simulink model "delay_complex_slr_test"  (Simulink 7.0)
settings: Solver=VariableStepDiscrete  StartTime=0.0  StopTime=500  RelTol=1e-3
libraries: xbsIndex_r4 x7, casper_library x6
settings Model: Creator=User  LastModifiedBy=User
settings DebuggingCC: SaveWithDisabledLinksMsg=none  SaveWithParameterizedLinksMsg=none

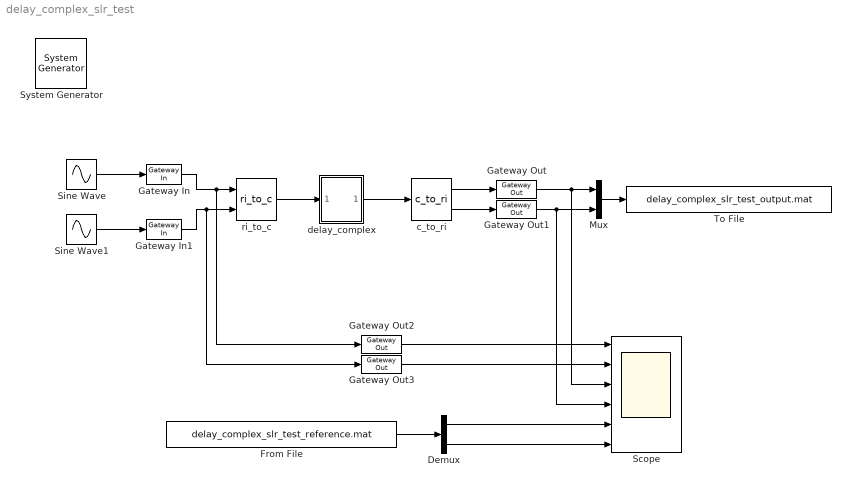
== system delay_complex_slr_test ==
  " System Generator" : xbsIndex_r4/ System Generator  Tag=genX  SystemSampleTime=-1  xilinxfamily=Virtex4  part=xc4vsx35  speed=-10  package=ff668  synthesis_tool=XST  clock_wrapper=Clock Enables  directory=./netlist  testbench=off  simulink_period=1  sysclk_period=100  dcm_input_clock_period=100  incr_netlist=off  trim_vbits=Everywhere in SubSystem  dbl_ovrd=According to Block Masks  core_generation=According to Block Masks  run_coregen=off  deprecated_control=off  eval_field=0  block_type=sysgen
      settings: block_version=10.1.1
  Demux : Demux  Outputs=2
  From File : FromFile  FileName=delay_complex_slr_test_reference.mat  SampleTime=1
  Gateway In : xbsIndex_r4/Gateway In  arith_type="Signed  (2's comp)"  n_bits=13  bin_pt=12  quantization=Truncate  overflow=Wrap  period=1  dbl_ovrd=off  timing_constraint=None  locs_specified=off  LOCs={}  block_type=gatewayin
      settings: infoedit="Gateway in block.  Converts inputs of type Simulink integer, double and fixed point to  Xilinx fixed point type.<P><P>Hardware notes:  In hardware these blocks become top level input ports."  block_version=10.1.1
  Gateway In1 : xbsIndex_r4/Gateway In  arith_type="Signed  (2's comp)"  n_bits=13  bin_pt=12  quantization=Truncate  overflow=Wrap  period=1  dbl_ovrd=off  timing_constraint=None  locs_specified=off  LOCs={}  block_type=gatewayin
      settings: infoedit="Gateway in block.  Converts inputs of type Simulink integer, double and fixed point to  Xilinx fixed point type.<P><P>Hardware notes:  In hardware these blocks become top level input ports."  block_version=10.1.1
  Gateway Out{,1..3} (4 alike) : xbsIndex_r4/Gateway Out  hdl_port=on  timing_constraint=None  locs_specified=off  LOCs={}  block_type=gatewayout
      settings: infoedit="Gateway out block.  Converts Xilinx fixed point inputs into ouputs of type Simulink integer, double, or fixed point.<P><P>Hardware notes:  In hardware these blocks become top level output ports or are discarded, depending on how they are configured."  block_version=10.1.1
  Mux : Mux  Inputs=2
  Scope : Scope  NumInputPorts=6
      settings: YMin=-5~-5~-5~-5~-5~-5  YMax=5~5~5~5~5~5
  Sine Wave : Sin  SineType=Sample based  SampleTime=1
  Sine Wave1 : Sin  SineType=Sample based  Samples=11  SampleTime=1  Offset=10
  To File : ToFile  Filename=delay_complex_slr_test_output.mat  MatrixName=output
  c_to_ri : casper_library/Misc/c_to_ri  SystemSampleTime=-1  n_bits=13  bin_pt=12
      settings: AttributesFormatString=13_12 r/i
  delay_complex : Subsystem  AncestorBlock=casper_library/Delays/delay_complex  mask(delay_complex){delay=7, n_bits=13, bin_pt=12, use_bram=0, bram_latency=4}
      mask prompts: delay "Delay Length"; n_bits "Sample Bit Width"; bin_pt "Binary Point"; use_bram "Use BRAM (0=no, 1=yes)"; bram_latency "BRAM Latency"
      mask help: A delay block that treats its input as complex, splits it into real and imaginary components, delays each component by a specified amount, and then re-joins them into a complex output. The underlying storage is user-selectable (either BRAM or SLR16 elements). The reason for this is wide (36 bit) delays make adjacent multipliers in multiplier-bram pairs unusable.
      mask init:
      | delay_complex_init(gcb, ...
      |     'delay', delay, ...
      |     'n_bits', n_bits, ...
      |     'bin_pt', bin_pt, ...
      |     'use_bram', use_bram, ...
      |     'bram_latency', bram_latency);
      settings: AttributesFormatString=|
      | depth = 7
      | delay_slr
      mask Help: eval('xlWeb([getenv(''MLIB_ROOT''), ''\doc\htmlblocks\sp_delay_complex\sp_delay_complex.html''])')
  ri_to_c : casper_library/Misc/ri_to_c  SystemSampleTime=-1
  wires:
  Sine Wave/1 -> Gateway In/1
  Sine Wave1/1 -> Gateway In1/1
  Gateway In/1 -> ri_to_c/1, Gateway Out2/1
  Gateway In1/1 -> ri_to_c/2, Gateway Out3/1
  ri_to_c/1 -> delay_complex/1(In1)
  c_to_ri/1 -> Gateway Out/1
  c_to_ri/2 -> Gateway Out1/1
  Gateway Out/1 -> Mux/1, Scope/3
  Gateway Out1/1 -> Mux/2, Scope/4
  Mux/1 -> To File/1
  delay_complex/1(Out1) -> c_to_ri/1
  Gateway Out2/1 -> Scope/1
  Gateway Out3/1 -> Scope/2
  From File/1 -> Demux/1
  Demux/1 -> Scope/5
  Demux/2 -> Scope/6

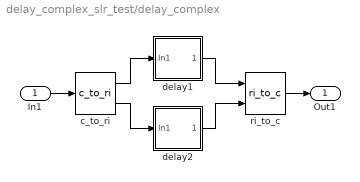
== system delay_complex_slr_test/delay_complex ==
  In1 : Inport  OutDataType=sfix(16)  OutScaling=2^0
  c_to_ri : casper_library/Misc/c_to_ri  SystemSampleTime=-1  n_bits=13  bin_pt=12
      settings: AttributesFormatString=13_12 r/i
  delay1 : Subsystem  BlockChoice=delay_slr
      link override delay_bram: DelayLen=delay  bram_latency=bram_latency
      link override delay_slr: DelayLen=delay
      settings: AttributesFormatString=%<BlockChoice>  TemplateBlock=casper_library/Delays/delay  MemberBlocks=delay_bram,delay_slr
  delay2 : Subsystem  BlockChoice=delay_slr
      link override delay_bram: DelayLen=delay  bram_latency=bram_latency
      link override delay_slr: DelayLen=delay
      settings: AttributesFormatString=%<BlockChoice>  TemplateBlock=casper_library/Delays/delay  MemberBlocks=delay_bram,delay_slr
  ri_to_c : casper_library/Misc/ri_to_c  SystemSampleTime=-1
  Out1 : Outport  OutDataType=sfix(16)  OutScaling=2^0
  wires:
  c_to_ri/1 -> delay1/1(In1)
  delay1/1(Out1) -> ri_to_c/1
  c_to_ri/2 -> delay2/1(In1)
  delay2/1(Out1) -> ri_to_c/2
  In1/1 -> c_to_ri/1
  ri_to_c/1 -> Out1/1

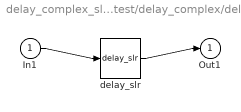
== system delay_complex_slr_test/delay_complex/delay1 ==
  In1 : Inport  OutDataType=sfix(16)  OutScaling=2^0
  delay_slr : casper_library/Delays/delay_slr  SystemSampleTime=-1  DelayLen=delay
  Out1 : Outport  OutDataType=sfix(16)  OutScaling=2^0
  wires:
  In1/1 -> delay_slr/1
  delay_slr/1 -> Out1/1

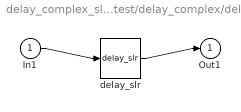
== system delay_complex_slr_test/delay_complex/delay2 ==
  In1 : Inport  OutDataType=sfix(16)  OutScaling=2^0
  delay_slr : casper_library/Delays/delay_slr  SystemSampleTime=-1  DelayLen=delay
  Out1 : Outport  OutDataType=sfix(16)  OutScaling=2^0
  wires:
  In1/1 -> delay_slr/1
  delay_slr/1 -> Out1/1
